simulink model "motor_mixer"  (R2016a)
settings: Solver=VariableStepAuto  StartTime=0.0  StopTime=10.0  RelTol=1e-3
settings Model: Creator=anne  LastModifiedBy=anne
settings GRTTargetCC: GeneratePreprocessorConditionals=Use local settings

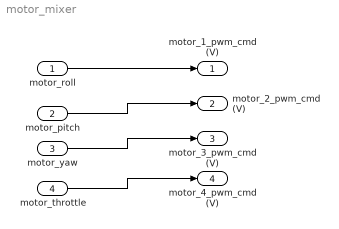
== system motor_mixer ==
  motor_roll : Inport
  motor_pitch : Inport  Port=2
  motor_yaw : Inport  Port=3
  motor_throttle : Inport  Port=4
  motor_1_pwm_cmd (V) : Outport
  motor_2_pwm_cmd (V) : Outport  Port=2
  motor_3_pwm_cmd (V) : Outport  Port=3
  motor_4_pwm_cmd (V) : Outport  Port=4
  wires:
  motor_roll/1 -> motor_1_pwm_cmd (V)/1
  motor_pitch/1 -> motor_2_pwm_cmd (V)/1
  motor_yaw/1 -> motor_3_pwm_cmd (V)/1
  motor_throttle/1 -> motor_4_pwm_cmd (V)/1
